simulink model "qpsk_transmitter"  (Simulink 6.6)
settings: Solver=ode45  StartTime=0.0  StopTime=0.1  RelTol=1e-3
PreLoadFcn:
  | rrc_weights
StopFcn:
  | figure(10)
  | hold off
  | plot(i_source(20:end),q_source(20:end),'bo','MarkerFaceColor','b','MarkerSize',6);
  | hold on
  | plot([0 0],[-1.5 1.5],'k:');
  | plot([-1.5 1.5],[0 0],'k:');
  | title('Constellation');
  | xlabel('In Phase');
  | ylabel('Quadrature');
  | axis([-1.5 1.5 -1.5 1.5]);
  | 
  | 
  | figure(11)
  | plot(tx_out);
  | title('Modulated QPSK Signal');
libraries: dsparch4 x2, dspsigops x2
settings Model: Creator=lcrockett  LastModifiedBy=lcrockett

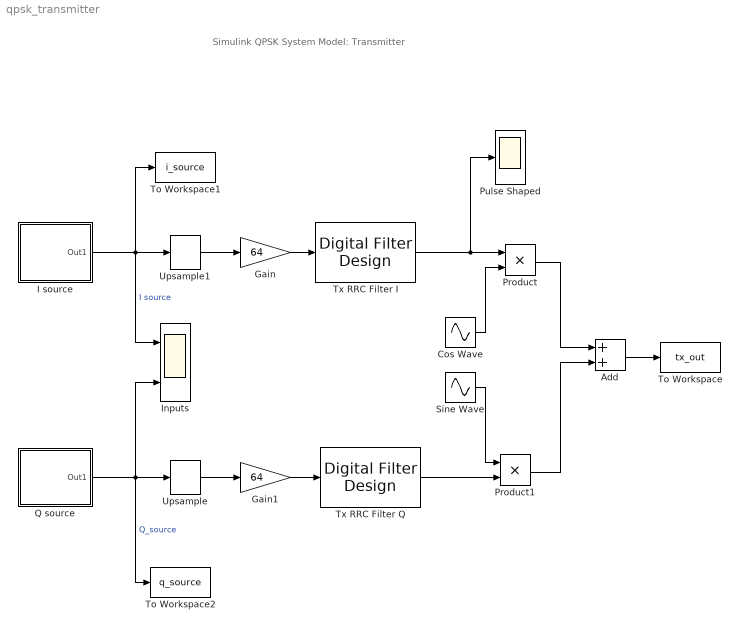
== system qpsk_transmitter ==
  note: Simulink QPSK System Model: Transmitter
  Add : Sum  OutScaling=2^-10
  Cos Wave : Sin  Frequency=(38.4e+3)*2*pi  Phase=pi/2  SampleTime=1/153.6e+3
  Gain : Gain  Gain=64
  Gain1 : Gain  Gain=64
  I source : Subsystem
  Inputs : Scope  NumInputPorts=2
      settings: YMin=-1.2~-1.2  YMax=1.2~1.2
  Product : Product  RndMeth=Zero
  Product1 : Product  RndMeth=Zero
  Pulse Shaped : Scope
      settings: YMin=-2  YMax=2
  Q source : Subsystem
  Sine Wave : Sin  Frequency=(38.4e+3)*2*pi  SampleTime=1/153.6e+3
  To Workspace : ToWorkspace  VariableName=tx_out  SampleTime=-1  SaveFormat=Array
  To Workspace1 : ToWorkspace  VariableName=i_source  SampleTime=-1  SaveFormat=Array
  To Workspace2 : ToWorkspace  VariableName=q_source  SampleTime=-1  SaveFormat=Array
  Tx RRC Filter I : dsparch4/Digital Filter Design  SystemSampleTime=-1  mwdsp_browser_bugfix_var=off
  Tx RRC Filter Q : dsparch4/Digital Filter Design  SystemSampleTime=-1  mwdsp_browser_bugfix_var=off
  Upsample : dspsigops/Upsample  N=64  phase=0  ic=0  mode=Maintain input frame size
  Upsample1 : dspsigops/Upsample  N=64  phase=0  ic=0  mode=Maintain input frame size
  wires:
  Q source/1(Out1) -> Upsample/1, Inputs/2, To Workspace2/1  "Q_source"
  Tx RRC Filter I/1 -> Product/1, Pulse Shaped/1
  Tx RRC Filter Q/1 -> Product1/2
  Product/1 -> Add/1
  Product1/1 -> Add/2
  Add/1 -> To Workspace/1
  Upsample/1 -> Gain1/1
  I source/1(Out1) -> Upsample1/1, Inputs/1, To Workspace1/1  "I source"
  Upsample1/1 -> Gain/1
  Sine Wave/1 -> Product1/1
  Cos Wave/1 -> Product/2
  Gain/1 -> Tx RRC Filter I/1
  Gain1/1 -> Tx RRC Filter Q/1

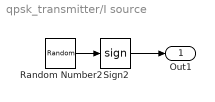
== system qpsk_transmitter/I source ==
  Random Number2 : RandomNumber  Seed=777  SampleTime=1/2400
  Sign2 : Signum
  Out1 : Outport
  wires:
  Random Number2/1 -> Sign2/1
  Sign2/1 -> Out1/1

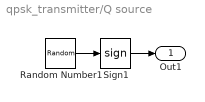
== system qpsk_transmitter/Q source ==
  Random Number1 : RandomNumber  Seed=99  SampleTime=1/2400
  Sign1 : Signum
  Out1 : Outport
  wires:
  Random Number1/1 -> Sign1/1
  Sign1/1 -> Out1/1
